simulink subsystem "HI_SPI"  (R2019b)
settings: Solver=VariableStepAuto  StartTime=0.0  StopTime=10.0  RelTol=1e-3
libraries: hdlsllib x2, c280xlib x2
settings Model: Creator=Nick  LastModifiedBy=zacha

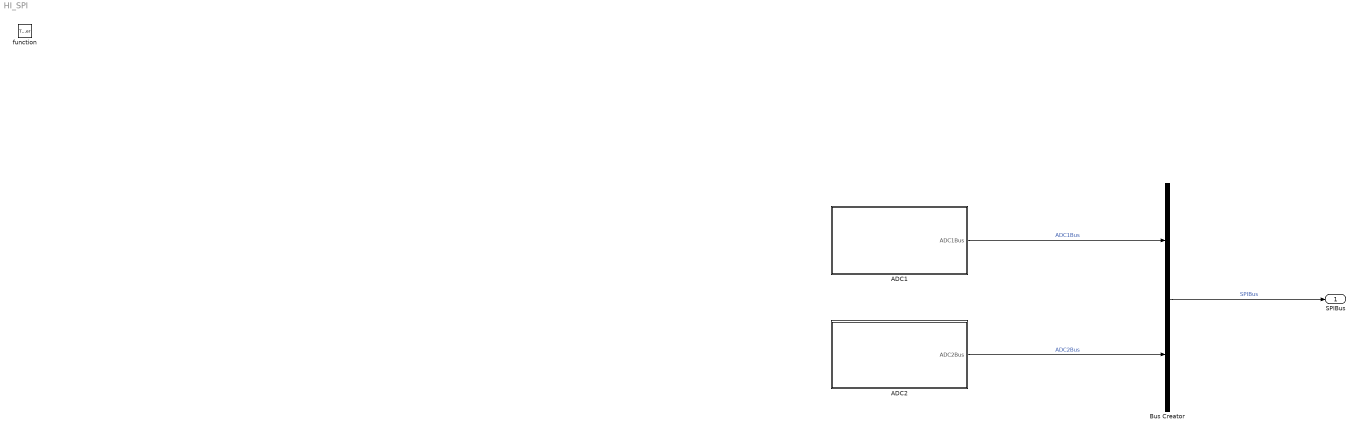
== system HI_SPI ==
  function : TriggerPort  TriggerType=function-call  VariantControl=Variant
  "ADC1 " : Subsystem
  ADC2 : Subsystem
  Bus Creator : BusCreator  Inputs=2
  SPIBus : Outport
  wires:
  Bus Creator/1 -> SPIBus/1  "SPIBus"
  "ADC1 "/1(ADC1Bus) -> Bus Creator/1  "ADC1Bus"
  ADC2/1(ADC2Bus) -> Bus Creator/2  "ADC2Bus"

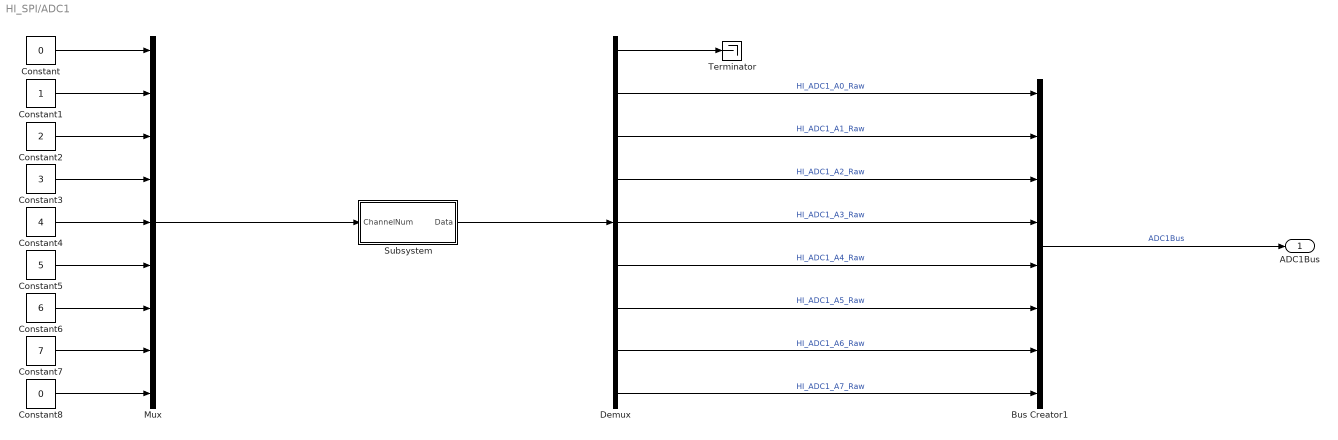
== system HI_SPI/ADC1  ==
  Bus Creator1 : BusCreator  Inputs=8
  Constant : Constant  Value=0
  Constant1 : Constant
  Constant2 : Constant  Value=2
  Constant3 : Constant  Value=3
  Constant4 : Constant  Value=4
  Constant5 : Constant  Value=5
  Constant6 : Constant  Value=6
  Constant7 : Constant  Value=7
  Constant8 : Constant  Value=0
  Demux : Demux  Outputs=9
  Mux : Mux  Inputs=9
  Subsystem : Subsystem
  Terminator : Terminator
  ADC1Bus : Outport
  wires:
  Bus Creator1/1 -> ADC1Bus/1  "ADC1Bus"
  Subsystem/1(Data) -> Demux/1
  Constant7/1 -> Mux/8
  Demux/8 -> Bus Creator1/7  "HI_ADC1_A6_Raw"
  Constant4/1 -> Mux/5
  Demux/3 -> Bus Creator1/2  "HI_ADC1_A1_Raw"
  Mux/1 -> Subsystem/1(ChannelNum)
  Demux/7 -> Bus Creator1/6  "HI_ADC1_A5_Raw"
  Demux/5 -> Bus Creator1/4  "HI_ADC1_A3_Raw"
  Constant8/1 -> Mux/9
  Demux/1 -> Terminator/1
  Constant1/1 -> Mux/2
  Constant/1 -> Mux/1
  Demux/9 -> Bus Creator1/8  "HI_ADC1_A7_Raw"
  Constant6/1 -> Mux/7
  Demux/4 -> Bus Creator1/3  "HI_ADC1_A2_Raw"
  Demux/6 -> Bus Creator1/5  "HI_ADC1_A4_Raw"
  Constant2/1 -> Mux/3
  Constant3/1 -> Mux/4
  Constant5/1 -> Mux/6
  Demux/2 -> Bus Creator1/1  "HI_ADC1_A0_Raw"

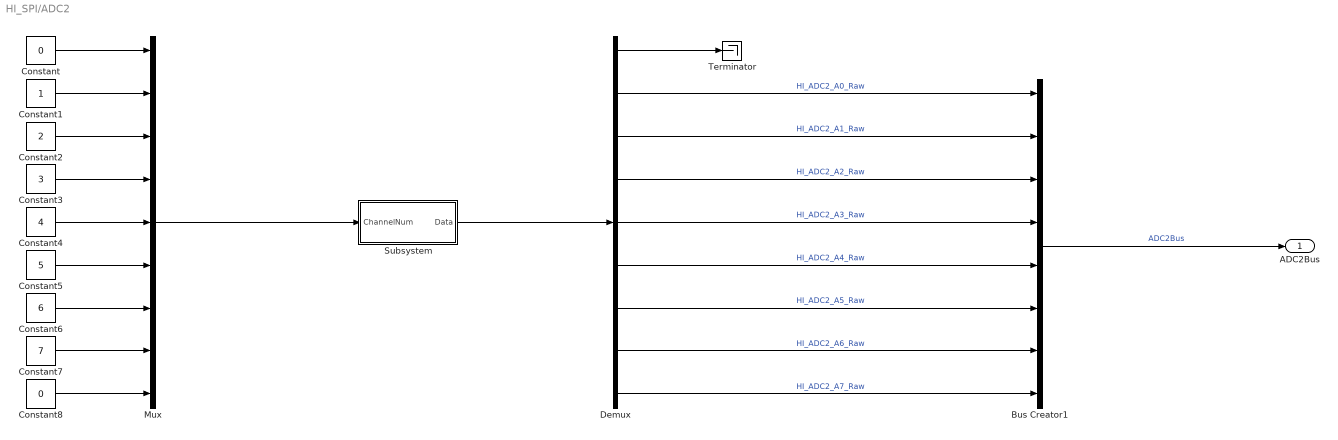
== system HI_SPI/ADC2 ==
  Bus Creator1 : BusCreator  Inputs=8
  Constant : Constant  Value=0
  Constant1 : Constant
  Constant2 : Constant  Value=2
  Constant3 : Constant  Value=3
  Constant4 : Constant  Value=4
  Constant5 : Constant  Value=5
  Constant6 : Constant  Value=6
  Constant7 : Constant  Value=7
  Constant8 : Constant  Value=0
  Demux : Demux  Outputs=9
  Mux : Mux  Inputs=9
  Subsystem : Subsystem
  Terminator : Terminator
  ADC2Bus : Outport
  wires:
  Bus Creator1/1 -> ADC2Bus/1  "ADC2Bus"
  Subsystem/1(Data) -> Demux/1
  Constant7/1 -> Mux/8
  Demux/8 -> Bus Creator1/7  "HI_ADC2_A6_Raw"
  Constant4/1 -> Mux/5
  Demux/3 -> Bus Creator1/2  "HI_ADC2_A1_Raw"
  Mux/1 -> Subsystem/1(ChannelNum)
  Demux/7 -> Bus Creator1/6  "HI_ADC2_A5_Raw"
  Demux/5 -> Bus Creator1/4  "HI_ADC2_A3_Raw"
  Constant8/1 -> Mux/9
  Demux/1 -> Terminator/1
  Constant1/1 -> Mux/2
  Constant/1 -> Mux/1
  Demux/9 -> Bus Creator1/8  "HI_ADC2_A7_Raw"
  Constant6/1 -> Mux/7
  Demux/4 -> Bus Creator1/3  "HI_ADC2_A2_Raw"
  Demux/6 -> Bus Creator1/5  "HI_ADC2_A4_Raw"
  Constant2/1 -> Mux/3
  Constant3/1 -> Mux/4
  Constant5/1 -> Mux/6
  Demux/2 -> Bus Creator1/1  "HI_ADC2_A0_Raw"

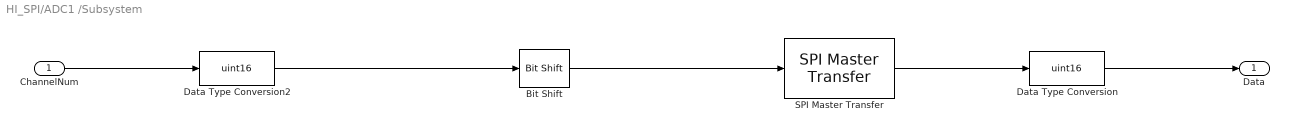
== system HI_SPI/ADC1 /Subsystem ==
  ChannelNum : Inport
  Bit Shift : hdlsllib/Logic and Bit Operations/Bit Shift  mode=Shift Left Logical  N=11
      settings: SourceProductName=Simulink
  Data Type Conversion : DataTypeConversion  OutDataTypeStr=uint16
  Data Type Conversion2 : DataTypeConversion  OutDataTypeStr=uint16
  SPI Master Transfer : c280xlib/SPI Master Transfer  SPISelect=SPI_A  ClockPolarity=Falling_edge  ClockPhase=No_delay  SPIModule=uint32(0)  Mode=Master  BusSpeed=uint32(1000000)  FirstBitToTransfer=Most significant bit (MSB)  ClockMode=0  BlockFunction=Transfer  EnableRegisterAddress=on  RegisterAddress=0  OutputDataType=int8  OutputDataLength=1  DataBits=16  UseCustomSSPin=Explicit GPIO calls  ActiveLowSSPin=Active low  Pin=3
      settings: SourceProductName=Embedded Coder Support Package for Texas Instruments C2000 Processors  SourceProductBaseCode=TIC2000
  Data : Outport
  wires:
  Bit Shift/1 -> SPI Master Transfer/1
  Data Type Conversion2/1 -> Bit Shift/1
  SPI Master Transfer/1 -> Data Type Conversion/1
  Data Type Conversion/1 -> Data/1
  ChannelNum/1 -> Data Type Conversion2/1

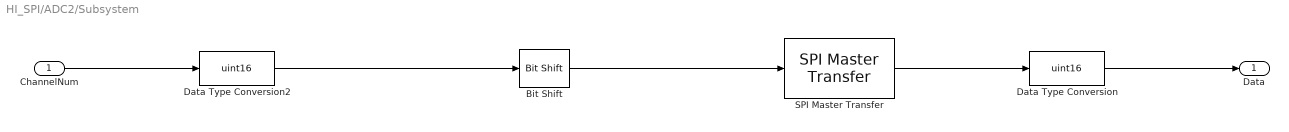
== system HI_SPI/ADC2/Subsystem ==
  ChannelNum : Inport
  Bit Shift : hdlsllib/Logic and Bit Operations/Bit Shift  mode=Shift Left Logical  N=11
      settings: SourceProductName=Simulink
  Data Type Conversion : DataTypeConversion  OutDataTypeStr=uint16
  Data Type Conversion2 : DataTypeConversion  OutDataTypeStr=uint16
  SPI Master Transfer : c280xlib/SPI Master Transfer  SPISelect=SPI_A  ClockPolarity=Falling_edge  ClockPhase=No_delay  SPIModule=uint32(0)  Mode=Master  BusSpeed=uint32(1000000)  FirstBitToTransfer=Most significant bit (MSB)  ClockMode=0  BlockFunction=Transfer  EnableRegisterAddress=on  RegisterAddress=0  OutputDataType=int8  OutputDataLength=1  DataBits=16  UseCustomSSPin=Explicit GPIO calls  ActiveLowSSPin=Active low  Pin=19
      settings: SourceProductName=Embedded Coder Support Package for Texas Instruments C2000 Processors  SourceProductBaseCode=TIC2000
  Data : Outport
  wires:
  Bit Shift/1 -> SPI Master Transfer/1
  Data Type Conversion2/1 -> Bit Shift/1
  SPI Master Transfer/1 -> Data Type Conversion/1
  Data Type Conversion/1 -> Data/1
  ChannelNum/1 -> Data Type Conversion2/1
